simulink model "simpleCounter"  (R2014a)
settings: Solver=FixedStepDiscrete  StartTime=0.0  StopTime=CONFIG.SIMULATION_TIME  FixedStep=CONFIG.Ts  RelTol=1e-3
InitFcn:
  | initSimpleCounter
values from neighbouring files (symbols this model uses):
  amplitude = 10    [initSimpleCounter.m]
  frequency = 3.5    [initSimpleCounter.m]
settings Model: Creator=gabri  LastModifiedBy=gabri
settings OptimizationCC: OptimizeModelRefInitCode=on  LifeSpan=1
settings RTWCC: SystemTargetFile=ert.tlc  TemplateMakefile=ert_default_tmf  Description=Embedded Coder  GenerateReport=on  ProcessScript=ert_make_rtw_hook  BuildConfiguration=Faster Runs  IncludeHyperlinkInReport=on  LaunchReport=on  TargetLang=C++
settings ERTTargetCC: TargetLangStandard=C++03 (ISO)  ParMdlRefBuildCompliant=on  CompOptLevelCompliant=on  ConcurrentExecutionCompliant=on  ERTFirstTimeCompliant=on  MultiInstanceERTCode=on  CodeInterfacePackaging=Reusable function  SupportContinuousTime=on  SupportNonInlinedSFcns=on  ModelStepFunctionPrototypeControlCompliant=on  CPPClassGenCompliant=on  InlinedParameterPlacement=Hierarchical  RootIOFormat=Structure reference  ERTCustomFileTemplate=example_file_process.tlc

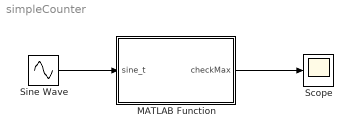
== system simpleCounter ==
  MATLAB Function : MATLAB Function  TreatAsAtomicUnit=on
  Scope : Scope
  Sine Wave : Sin  Amplitude=amplitude  Frequency=frequency  SampleTime=0
  wires:
  Sine Wave/1 -> MATLAB Function/1(sine_t)
  MATLAB Function/1(checkMax) -> Scope/1

== matlab function simpleCounter/MATLAB Function ==
  data: sine_t input; checkMax output; amplitude parameter
function checkMax = fcn(sine_t,amplitude)

    % just check if sine_t = amplitude. Returns 0 otherwise. 
    checkMax = 0;
    toll     = 0.01;

    if sine_t >= amplitude-toll
        checkMax = 1;
    end
end
